simulink model "part_01"  (R2022b)
settings: Solver=VariableStepAuto  StartTime=0.0  StopTime=10.0  RelTol=1e-3
undefined symbols (not defined in the file): j, kd, T
settings Model: Creator=Admin  LastModifiedBy=Admin

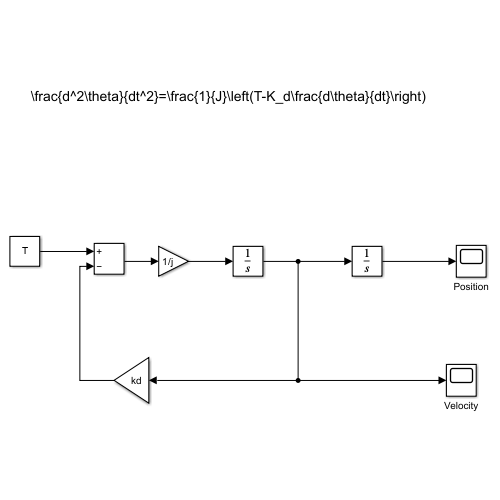
[thumbnail: Simulink's stored preview of the top-level diagram]
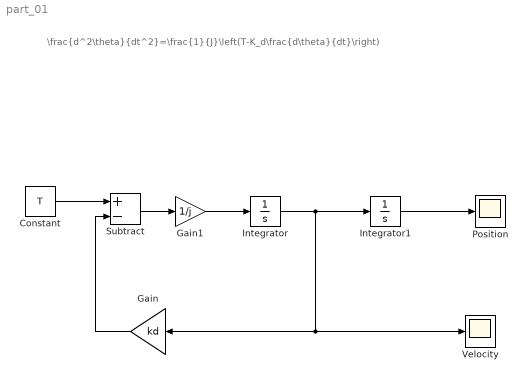
== system part_01 ==
  note: \frac{d^2\theta}{dt^2}=\frac{1}{J}\left(T-K_d\frac{d\theta}{dt}\right)
  Constant : Constant  Value=T
  Gain : Gain  Gain=kd
  Gain1 : Gain  Gain=1/j
  Integrator : Integrator
  Integrator1 : Integrator
  Position : Scope
  Subtract : Sum  Inputs=+-
  Velocity : Scope
  wires:
  Integrator1/1 -> Position/1
  Integrator/1 -> Gain/1, Velocity/1, Integrator1/1
  Gain1/1 -> Integrator/1
  Constant/1 -> Subtract/1
  Subtract/1 -> Gain1/1
  Gain/1 -> Subtract/2
